simulink model "nmm2DFullBody"  (R2015b)
settings: Solver=ode23s  StartTime=0.0  StopTime=13  FixedStep=1e-3  MaxStep=ts_max  RelTol=1e-3  AbsTol=1e-4
InitFcn:
  | addpath('../lib');
  | addpath('./init_script');
  | nms_model_MechInit
  | nms_model_ControlInit
StopFcn:
  | mRFX = struct;
  | 
  | mRFX.RStance = DataFromModel.Data(:,2)
  | mRFX.RGRF_AP = DataFromModel.Data(:,24)
  | mRFX.RGRF_VT = DataFromModel.Data(:,22)
  | mRFX.RAnkleAngle = DataFromModel.Data(:,8)
  | mRFX.RKneeAngle = DataFromModel.Data(:,7)
  | mRFX.RHipAngle = DataFromModel.Data(:,6)
  | mRFX.RAnkleTorque = DataFromModel.Data(:,20)
  | mRFX.RKneeTorque = DataFromModel.Data(:,19)
  | mRFX.RHipTorque = DataFromModel.Data(:,18)
  | 
  | mRFX.RMuscleGLU = DataFromModel.Data(:,32)
  | mRFX.RMuscleHF = DataFromModel.Data(:,33)
  | mRFX.RMuscleHAM = DataFromModel.Data(:,34)
  | mRFX.RMuscleVAS = DataFromModel.Data(:,35)
  | mRFX.RMuscleGAS = DataFromModel.Data(:,36)
  | mRFX.RMuscleSOL = DataFromModel.Data(:,37)
  | mRFX.RMuscleTA = DataFromModel.Data(:,38)
  | 
  | mRFX.LStance = DataFromModel.Data(:,1)
  | mRFX.LGRF_AP = DataFromModel.Data(:,23)
  | mRFX.LGRF_VT = DataFromModel.Data(:,21)
  | mRFX.LAnkleAngle = DataFromModel.Data(:,5)
  | mRFX.LKneeAngle = DataFromModel.Data(:,4)
  | mRFX.LHipAngle = DataFromModel.Data(:,3)
  | mRFX.LAnkleTorque = DataFromModel.Data(:,17)
  | mRFX.LKneeTorque = DataFromModel.Data(:,16)
  | mRFX.LHipTorque = DataFromModel.Data(:,15)
  | 
  | mRFX.LMuscleGLU = DataFromModel.Data(:,25)
  | mRFX.LMuscleHF = DataFromModel.Data(:,26)
  | mRFX.LMuscleHAM = DataFromModel.Data(:,27)
  | mRFX.LMuscleVAS = DataFromModel.Data(:,28)
  | mRFX.LMuscleGAS = DataFromModel.Data(:,29)
  | mRFX.LMuscleSOL = DataFromModel.Data(:,30)
  | mRFX.LMuscleTA = DataFromModel.Data(:,31)
values from neighbouring files (symbols this model uses):
  c = load('struct_mRFX_HAM_symetric_feedback.mat')    [Ex2b.m]
undefined symbols (not defined in the file or in its folder): alphaFmGas, alphaFmGlu, alphaFmHam, alphaFmSol, alphaFmVas, alphaLceHam, alphaLceHfl, alphaLceTa, alphaLceTa1, Amp, amp_var, c_jointstop, D12_F, D12_S, D12_T, D13_F, D1G_F, D1G_HAT, D1G_S, D1G_T, DeltaThRef, eref, FmaxGAS, FmaxGLU, FmaxHAM, FmaxHFL, FmaxSOL, FmaxTA, FmaxVAS, freq, freq_var, GainDeltaTheta, GainGAS, GainGLU, GainHAM, GainHAMHFL, GainHFL, GainKneOverExt, GainSOL, GainSOLTA, GainTA, GainVAS, In_F, In_HAT, In_S, In_T, K, k_gx, k_gy, k_pressure, K_swing, LceOffsetHAM, LceOffsetHFL, LceOffsetTA, LongDelay, loptGAS, loptGLU, loptHAM, loptHFL, loptSOL ... (+82)
libraries: nmc x77, mblibv1 x60, simulink x33, simulink_extras x18
(part 4 of 8)

== system nmm2DFullBody/Full Body Control (created using the nmc library)/Left Side/HFL&HAM Muscles/HAM Actuation  ==
  note: HAM Actuation
  phiHip : Inport
  phiKnee : Inport  Port=2
  StimHam : Inport  Port=3
  " HAM Muscle Spindles" : Gain  Gain=1/loptHAM
  " HAM Fm loop delay" : TransportDelay  DelayTime=ShortDelay
  " HAM Link" : Subsystem
  HAM : Subsystem
  HAM Golgi Tendon Organs : Gain
  HAM Lce loop delay : TransportDelay  DelayTime=ShortDelay
  Mux1 : Mux  Inputs=5
  Product8 : Product  RndMeth=Zero
  Product9 : Product  RndMeth=Zero
  Saturation7 : Saturate  UpperLimit=inf  LowerLimit=0  ZeroCross=off
  Stimulation Bias7 : Constant  Value=LceOffsetHAM
  Subsystem3 : nmc/Subsystem4  GotoTag=LEFT_HAM_FORCE  GotoTag2=LEFT_HAM_FORCE_LOG  GotoTag3=LEFT_HAM_FORCE_NOISE_LOG
  Subsystem5 : nmc/Subsystem4  GotoTag=LEFT_HAM_STIM  GotoTag2=LEFT_HAM_STIM_LOG  GotoTag3=LEFT_HAM_STIM_NOISE_LOG
  Subsystem6 : nmc/Subsystem4  GotoTag=LEFT_HAM_LENGTH  GotoTag2=LEFT_HAM_LENGTH_LOG  GotoTag3=LEFT_HAM_LENGTH_NOISE_LOG
  Subsystem7 : nmc/Subsystem4  GotoTag=LEFT_HAM_VELOCITY  GotoTag2=LEFT_HAM_VELOCITY_LOG  GotoTag3=LEFT_HAM_VELOCITY_NOISE_LOG
  Subsystem8 : nmc/Subsystem4  GotoTag=LEFT_HAM_GOLGI  GotoTag2=LEFT_HAM_GOLGI_LOG  GotoTag3=LEFT_HAM_GOLGI_NOISE_LOG
  Sum26 : Sum  Inputs=-+|  SaturateOnIntegerOverflow=on  InputSameDT=on  OutDataTypeStr=Inherit: Same as first input
  Terminator1 : Terminator
  TauHamHip : Outport
  TauHamKnee : Outport  Port=2
  LceHam : Outport  Port=3
  FmHam : Outport  Port=4
  wires:
  phiKnee/1 -> " HAM Link"/2(phi23 [rad])
  HAM/1(Fmtc) -> Subsystem3/1
  HAM/2(Lce) -> Subsystem6/1
  " HAM Link"/2(lever34 [m]) -> Product8/2
  " HAM Link"/3(lever23 [m]) -> Product9/2
  phiHip/1 -> " HAM Link"/1(phi34 [rad])
  HAM/5(A) -> Mux1/5
  Product8/1 -> TauHamHip/1
  HAM Golgi Tendon Organs/1 -> " HAM Fm loop delay"/1
  " HAM Muscle Spindles"/1 -> Sum26/2
  Sum26/1 -> Saturation7/1
  Mux1/1 -> Terminator1/1
  HAM/4(Lse) -> Mux1/4
  HAM/3(Vce) -> Subsystem7/1
  Stimulation Bias7/1 -> Sum26/1
  Product9/1 -> TauHamKnee/1
  StimHam/1 -> Subsystem5/1
  Saturation7/1 -> HAM Lce loop delay/1
  HAM Lce loop delay/1 -> LceHam/1
  " HAM Fm loop delay"/1 -> FmHam/1
  Subsystem3/1 -> Mux1/1, Subsystem8/1, Product9/1, Product8/1
  Subsystem6/1 -> " HAM Muscle Spindles"/1, Mux1/2
  Subsystem7/1 -> Mux1/3
  " HAM Link"/1(lmtu [m]) -> HAM/2(lmtc [m])
  Subsystem5/1 -> HAM/1(STIM)
  Subsystem8/1 -> HAM Golgi Tendon Organs/1

== system nmm2DFullBody/Full Body Control (created using the nmc library)/Left Side/HFL&HAM Muscles/HFL Actuation ==
  note: HFL Actuation
  phiHip : Inport
  StimHFL : Inport  Port=2
  " HFL" : Subsystem
  " HFL Muscle Spindles" : Gain  Gain=1/loptHFL
  " HFL Link" : Subsystem
  Gain : Gain  Gain=-1
  HFL Lce loop delay : TransportDelay  DelayTime=ShortDelay
  Mux10 : Mux  Inputs=5
  Product7 : Product  RndMeth=Zero
  Saturation5 : Saturate  UpperLimit=inf  LowerLimit=0  ZeroCross=off
  Stimulation Bias5 : Constant  Value=LceOffsetHFL
  Subsystem3 : nmc/Subsystem4  GotoTag=LEFT_HF_FORCE  GotoTag2=LEFT_HF_FORCE_LOG  GotoTag3=LEFT_HF_FORCE_NOISE_LOG
  Subsystem5 : nmc/Subsystem4  GotoTag=LEFT_HF_STIM  GotoTag2=LEFT_HF_STIM_LOG  GotoTag3=LEFT_HF_STIM_NOISE_LOG
  Subsystem6 : nmc/Subsystem4  GotoTag=LEFT_HF_LENGTH  GotoTag2=LEFT_HF_LENGTH_LOG  GotoTag3=LEFT_HF_LENGTH_NOISE_LOG
  Subsystem7 : nmc/Subsystem4  GotoTag=LEFT_HF_VELOCITY  GotoTag2=LEFT_HF_VELOCITY_LOG  GotoTag3=LEFT_HF_VELOCITY_NOISE_LOG
  Sum24 : Sum  Inputs=-+|  SaturateOnIntegerOverflow=on  InputSameDT=on  OutDataTypeStr=Inherit: Same as first input
  Terminator10 : Terminator
  TauHFL : Outport
  LceHFL : Outport  Port=2
  wires:
  Stimulation Bias5/1 -> Sum24/1
  " HFL"/1(Fmtc) -> Subsystem3/1
  " HFL"/2(Lce) -> Subsystem6/1
  " HFL Link"/1(lmtu [m]) -> " HFL"/2(lmtc [m])
  " HFL"/5(A) -> Mux10/5
  " HFL Link"/2(lever [m]) -> Product7/1
  " HFL Muscle Spindles"/1 -> Sum24/2
  Sum24/1 -> Saturation5/1
  Saturation5/1 -> HFL Lce loop delay/1
  Mux10/1 -> Terminator10/1
  " HFL"/4(Lse) -> Mux10/4
  " HFL"/3(Vce) -> Subsystem7/1
  phiHip/1 -> " HFL Link"/1(phi34 [rad])
  StimHFL/1 -> Subsystem5/1
  Product7/1 -> Gain/1
  Gain/1 -> TauHFL/1
  HFL Lce loop delay/1 -> LceHFL/1
  Subsystem5/1 -> " HFL"/1(STIM)
  Subsystem6/1 -> " HFL Muscle Spindles"/1, Mux10/2
  Subsystem7/1 -> Mux10/3
  Subsystem3/1 -> Product7/2, Mux10/1

== system nmm2DFullBody/Full Body Control (created using the nmc library)/Left Side/HFL&HAM Muscles/HFL&HAM Control ==
  note: HFL with HAM Control
  LceHFL : Inport
  LceHam : Inport  Port=2
  FmHam : Inport  Port=3
  Theta : Inport  Port=4
  dTheta : Inport  Port=5
  CLdxThigh : Inport  Port=6
  OLonCL : Inport  Port=7
  StanceSwing : Inport  Port=8
  "ANMC STIM " : Concatenate  NumInputs=1
  ANMC STIM 1 : Concatenate  NumInputs=1
  Demux : Demux  Outputs=2
  Logical Operator : Logic  Operator=NOT  AllPortsSameDT=off  OutDataTypeStr=boolean
  Mux1 : Mux  Inputs=2
  Mux2 : Mux  Inputs=2
  Saturation17 : Saturate  UpperLimit=1  LowerLimit=0.01  ZeroCross=off
  Stance Phase : Subsystem  TreatAsAtomicUnit=on
  Sum18 : Sum
  Swing Phase : Subsystem  TreatAsAtomicUnit=on
  StimHFL : Outport
  StimHAM : Outport  Port=2
  wires:
  Logical Operator/1 -> Swing Phase/Enable
  Theta/1 -> Stance Phase/1(Theta)
  dTheta/1 -> Stance Phase/2(dTheta [rad/s])
  Swing Phase/1(StimHFL) -> Mux1/1
  LceHam/1 -> Swing Phase/3(LceHAM)
  FmHam/1 -> Swing Phase/4(FmHAM)
  Stance Phase/3(Delta_Theta) -> Swing Phase/1(Delta_Theta)
  CLdxThigh/1 -> Stance Phase/3(CLdxThigh [N])
  Stance Phase/1(StimHFL) -> Mux2/1
  Stance Phase/2(StimHAM) -> Mux2/2
  LceHFL/1 -> Swing Phase/2(LceHFL)
  StanceSwing/1 -> Stance Phase/Enable, Logical Operator/1
  Sum18/1 -> Saturation17/1
  Saturation17/1 -> Demux/1
  Mux2/1 -> Sum18/1
  Mux1/1 -> Sum18/2
  Swing Phase/2(StimHAM) -> Mux1/2
  OLonCL/1 -> Stance Phase/4(OLonCL)
  Demux/2 -> ANMC STIM 1/1
  Demux/1 -> "ANMC STIM "/1
  "ANMC STIM "/1 -> StimHFL/1
  ANMC STIM 1/1 -> StimHAM/1

== system nmm2DFullBody/Full Body Control (created using the nmc library)/Left Side/HipJoint left/Hip Joint Limits ==
  note: Hip Joint Limits
  phi [rad] : Inport
  dphi [rad/s] : Inport  Port=2
  Gain2 : Gain  Gain=-1
  Gain3 : Gain  Gain=c_jointstop
  Gain4 : Gain  Gain=1/w_max_jointstop
  Limit Hip Range : simulink/Logic and Bit Operations/Interval Test  IntervalClosedRight=on  uplimit=phi34_UpLimit + 30*pi/180  IntervalClosedLeft=on  lowlimit=10*pi/180  OutDataTypeStr=boolean
  Logical Operator3 : Logic  Operator=NOT  AllPortsSameDT=off  OutDataTypeStr=boolean
  Mux3 : Mux  Inputs=2
  Overextension Torque : Fcn  Expr="- u(1)  *  (1-u(2)) * (u(2)<1) * (u(1)>0)"
  Stop Simulation1 : Stop
  Sum : Sum  Inputs=|+-
  overextension angle : Constant  Value=phi34_UpLimit
  M_stop [Nm] : Outport
  wires:
  Mux3/1 -> Overextension Torque/1
  Gain3/1 -> Mux3/1
  dphi [rad/s]/1 -> Gain4/1
  overextension angle/1 -> Sum/2
  phi [rad]/1 -> Sum/1, Limit Hip Range/1
  Sum/1 -> Gain3/1
  Gain4/1 -> Gain2/1
  Gain2/1 -> Mux3/2
  Overextension Torque/1 -> M_stop [Nm]/1
  Limit Hip Range/1 -> Logical Operator3/1
  Logical Operator3/1 -> Stop Simulation1/1

== system nmm2DFullBody/Full Body Control (created using the nmc library)/Left Side/KneeJoint left/Knee Joint Limits ==
  note: Knee Joint Limits
  phi [rad] : Inport
  dphi [rad/s] : Inport  Port=2
  Gain2 : Gain  Gain=-1
  Gain3 : Gain  Gain=c_jointstop
  Gain4 : Gain  Gain=1/w_max_jointstop
  Limit Knee Range : simulink/Logic and Bit Operations/Interval Test  IntervalClosedRight=on  uplimit=185*pi/180  IntervalClosedLeft=on  lowlimit=40*pi/180  OutDataTypeStr=boolean
  Logical Operator3 : Logic  Operator=NOT  AllPortsSameDT=off  OutDataTypeStr=boolean
  Mux3 : Mux  Inputs=2
  Overextension Torque : Fcn  Expr="- u(1)  *  (1-u(2)) * (u(2)<1) * (u(1)>0)"
  Stop Simulation1 : Stop
  Sum : Sum  Inputs=|+-
  overextension angle : Constant  Value=phi23_UpLimit
  M_stop [Nm] : Outport
  wires:
  Mux3/1 -> Overextension Torque/1
  Gain3/1 -> Mux3/1
  dphi [rad/s]/1 -> Gain4/1
  overextension angle/1 -> Sum/2
  phi [rad]/1 -> Sum/1, Limit Knee Range/1
  Sum/1 -> Gain3/1
  Gain4/1 -> Gain2/1
  Gain2/1 -> Mux3/2
  Overextension Torque/1 -> M_stop [Nm]/1
  Limit Knee Range/1 -> Logical Operator3/1
  Logical Operator3/1 -> Stop Simulation1/1

== system nmm2DFullBody/Full Body Control (created using the nmc library)/Left Side/SOL&TA Muscles/SOL Actuation ==
  note: SOL Actuation
  phiAnkle : Inport
  StimSOL : Inport  Port=2
  " SOL" : Subsystem
  " SOL Golgi Tendon Organs" : Gain
  Mux3 : Mux  Inputs=5
  Product : Product  RndMeth=Zero
  SOL Link : Subsystem
  SOL loop delay : TransportDelay  DelayTime=LongDelay
  Subsystem3 : nmc/Subsystem4  GotoTag=LEFT_SOL_FORCE  GotoTag2=LEFT_SOL_FORCE_LOG  GotoTag3=LEFT_SOL_FORCE_NOISE_LOG
  Subsystem5 : nmc/Subsystem4  GotoTag=LEFT_SOL_STIM  GotoTag2=LEFT_SOL_STIM_LOG  GotoTag3=LEFT_SOL_STIM_NOISE_LOG
  Subsystem6 : nmc/Subsystem4  GotoTag=LEFT_SOL_LENGTH  GotoTag2=LEFT_SOL_LENGTH_LOG  GotoTag3=LEFT_SOL_LENGTH_NOISE_LOG
  Subsystem7 : nmc/Subsystem4  GotoTag=LEFT_SOL_VELOCITY  GotoTag2=LEFT_SOL_VELOCITY_LOG  GotoTag3=LEFT_SOL_VELOCITY_NOISE_LOG
  Subsystem8 : nmc/Subsystem4  GotoTag=LEFT_SOL_GOLGI  GotoTag2=LEFT_SOL_GOLGI_LOG  GotoTag3=LEFT_SOL_GOLGI_NOISE_LOG
  Terminator3 : Terminator
  TauSOL : Outport
  FmSOL : Outport  Port=2
  wires:
  " SOL"/1(Fmtc) -> Subsystem3/1
  SOL Link/1(lmtc [m]) -> " SOL"/2(lmtc [m])
  SOL Link/2(lever [m]) -> Product/1
  Product/1 -> TauSOL/1
  " SOL"/5(A) -> Mux3/5
  Mux3/1 -> Terminator3/1
  " SOL"/2(Lce) -> Subsystem6/1
  " SOL"/3(Vce) -> Subsystem7/1
  " SOL"/4(Lse) -> Mux3/4
  phiAnkle/1 -> SOL Link/1(phi12 [rad])
  StimSOL/1 -> Subsystem5/1
  " SOL Golgi Tendon Organs"/1 -> SOL loop delay/1
  SOL loop delay/1 -> FmSOL/1
  Subsystem5/1 -> " SOL"/1(STIM)
  Subsystem3/1 -> Mux3/1, Product/2, Subsystem8/1
  Subsystem6/1 -> Mux3/2
  Subsystem7/1 -> Mux3/3
  Subsystem8/1 -> " SOL Golgi Tendon Organs"/1

== system nmm2DFullBody/Full Body Control (created using the nmc library)/Left Side/SOL&TA Muscles/SOL&TA Control ==
  note: SOL with TA Control
  LceTA : Inport
  FmSOL : Inport  Port=2
  StanceSwing : Inport  Port=3
  " Stance Phase" : Subsystem  TreatAsAtomicUnit=on
  "ANMC STIM " : Concatenate  NumInputs=1
  ANMC STIM 1 : Concatenate  NumInputs=1
  Demux : Demux  Outputs=2
  Logical Operator : Logic  Operator=NOT  AllPortsSameDT=off  OutDataTypeStr=boolean
  Mux1 : Mux  Inputs=2
  Mux2 : Mux  Inputs=2
  Saturation17 : Saturate  UpperLimit=1  LowerLimit=0.01  ZeroCross=off
  Sum18 : Sum
  Swing Phase : Subsystem  TreatAsAtomicUnit=on
  StimTA : Outport
  StimSOL : Outport  Port=2
  wires:
  Logical Operator/1 -> Swing Phase/Enable
  FmSOL/1 -> " Stance Phase"/1(FmSOL)
  StanceSwing/1 -> " Stance Phase"/Enable, Logical Operator/1
  LceTA/1 -> Swing Phase/1(LceTA), " Stance Phase"/2(LceTA)
  Swing Phase/1(StimTA) -> Mux1/1
  " Stance Phase"/1(StimTA) -> Mux2/1
  " Stance Phase"/2(StimSOL) -> Mux2/2
  Sum18/1 -> Saturation17/1
  Saturation17/1 -> Demux/1
  Mux2/1 -> Sum18/1
  Mux1/1 -> Sum18/2
  Swing Phase/2(StimSOL) -> Mux1/2
  Demux/2 -> ANMC STIM 1/1
  Demux/1 -> "ANMC STIM "/1
  "ANMC STIM "/1 -> StimTA/1
  ANMC STIM 1/1 -> StimSOL/1

== system nmm2DFullBody/Full Body Control (created using the nmc library)/Left Side/SOL&TA Muscles/TA Actuation ==
  note: TA Actuation
  phiAnkle : Inport
  StimTA : Inport  Port=2
  " TA Muscle Spindles" : Gain  Gain=1/loptTA
  " TA loop delay" : TransportDelay  DelayTime=LongDelay
  Gain : Gain  Gain=-1
  Mux8 : Mux  Inputs=5
  Product1 : Product  RndMeth=Zero
  Saturation2 : Saturate  UpperLimit=inf  LowerLimit=0  ZeroCross=off
  Stimulation Bias3 : Constant  Value=LceOffsetTA
  Subsystem3 : nmc/Subsystem4  GotoTag=LEFT_TA_FORCE  GotoTag2=LEFT_TA_FORCE_LOG  GotoTag3=LEFT_TA_FORCE_NOISE_LOG
  Subsystem5 : nmc/Subsystem4  GotoTag=LEFT_TA_STIM  GotoTag2=LEFT_TA_STIM_LOG  GotoTag3=LEFT_TA_STIM_NOISE_LOG
  Subsystem6 : nmc/Subsystem4  GotoTag=LEFT_TA_LENGTH  GotoTag2=LEFT_TA_LENGTH_LOG  GotoTag3=LEFT_TA_LENGTH_NOISE_LOG
  Subsystem7 : nmc/Subsystem4  GotoTag=LEFT_TA_VELOCITY  GotoTag2=LEFT_TA_VELOCITY_LOG  GotoTag3=LEFT_TA_VELOCITY_NOISE_LOG
  Sum21 : Sum  Inputs=-+|  SaturateOnIntegerOverflow=on  InputSameDT=on  OutDataTypeStr=Inherit: Same as first input
  TA : Subsystem
  TA Link : Subsystem
  Terminator8 : Terminator
  LceTA : Outport
  TauTa : Outport  Port=2
  wires:
  TA/1(Fmtc) -> Subsystem3/1
  TA/2(Lce) -> Subsystem6/1
  TA/5(A) -> Mux8/5
  TA Link/1(lmtc [m]) -> TA/2(lmtc [m])
  TA Link/2(lever [m]) -> Product1/2
  " TA Muscle Spindles"/1 -> Sum21/2
  Sum21/1 -> Saturation2/1
  Mux8/1 -> Terminator8/1
  TA/4(Lse) -> Mux8/4
  TA/3(Vce) -> Subsystem7/1
  phiAnkle/1 -> TA Link/1(phi12 [rad])
  Stimulation Bias3/1 -> Sum21/1
  Saturation2/1 -> " TA loop delay"/1
  Product1/1 -> Gain/1
  StimTA/1 -> Subsystem5/1
  " TA loop delay"/1 -> LceTA/1
  Gain/1 -> TauTa/1
  Subsystem5/1 -> TA/1(STIM)
  Subsystem3/1 -> Product1/1, Mux8/1
  Subsystem6/1 -> " TA Muscle Spindles"/1, Mux8/2
  Subsystem7/1 -> Mux8/3

== system nmm2DFullBody/Full Body Control (created using the nmc library)/Left Side/VAS Muscle/VAS Actuation  ==
  note: VAS Actuation
  phiKnee : Inport
  StimVas : Inport  Port=2
  " VAS Golgi Tendon Organs" : Gain
  Gain : Gain  Gain=-1
  Mux9 : Mux  Inputs=5
  Product4 : Product  RndMeth=Zero
  Subsystem3 : nmc/Subsystem4  GotoTag=LEFT_VAS_FORCE  GotoTag2=LEFT_VAS_FORCE_LOG  GotoTag3=LEFT_VAS_FORCE_NOISE_LOG
  Subsystem5 : nmc/Subsystem4  GotoTag=LEFT_VAS_STIM  GotoTag2=LEFT_VAS_STIM_LOG  GotoTag3=LEFT_VAS_STIM_NOISE_LOG
  Subsystem6 : nmc/Subsystem4  GotoTag=LEFT_VAS_LENGTH  GotoTag2=LEFT_VAS_LENGTH_LOG  GotoTag3=LEFT_VAS_LENGTH_NOISE_LOG
  Subsystem7 : nmc/Subsystem4  GotoTag=LEFT_VAS_VELOCITY  GotoTag2=LEFT_VAS_VELOCITY_LOG  GotoTag3=LEFT_VAS_VELOCITY_NOISE_LOG
  Subsystem8 : nmc/Subsystem4  GotoTag=LEFT_VAS_GOLGI  GotoTag2=LEFT_VAS_GOLGI_LOG  GotoTag3=LEFT_VAS_GOLGI_NOISE_LOG
  Terminator9 : Terminator
  VAS : Subsystem
  VAS Link : Subsystem
  VAS loop delay : TransportDelay  DelayTime=MidDelay
  TauVas : Outport
  FmVas : Outport  Port=2
  wires:
  Product4/1 -> Gain/1
  VAS/5(A) -> Mux9/5
  VAS/1(Fmtc) -> Subsystem3/1
  VAS Link/2(lever [m]) -> Product4/1
  Mux9/1 -> Terminator9/1
  VAS/4(Lse) -> Mux9/4
  VAS/3(Vce) -> Subsystem7/1
  VAS/2(Lce) -> Subsystem6/1
  phiKnee/1 -> VAS Link/1(phi23 [rad])
  StimVas/1 -> Subsystem5/1
  Gain/1 -> TauVas/1
  " VAS Golgi Tendon Organs"/1 -> VAS loop delay/1
  VAS loop delay/1 -> FmVas/1
  VAS Link/1(lmtu [m]) -> VAS/2(lmtc [m])
  Subsystem3/1 -> Subsystem8/1, Product4/2, Mux9/1
  Subsystem6/1 -> Mux9/2
  Subsystem7/1 -> Mux9/3
  Subsystem5/1 -> VAS/1(STIM)
  Subsystem8/1 -> " VAS Golgi Tendon Organs"/1

== system nmm2DFullBody/Full Body Control (created using the nmc library)/Left Side/VAS Muscle/VAS Control ==
  note: VAS Control
  FmVAS : Inport
  OLdxThigh : Inport  Port=2
  OLonCL : Inport  Port=3
  CLKneeState : Inport  Port=4
  StanceSwing : Inport  Port=5
  " Swing Phase" : Subsystem  TreatAsAtomicUnit=on
  "ANMC STIM " : Concatenate  NumInputs=1
  Logical Operator : Logic  Operator=NOT  AllPortsSameDT=off  OutDataTypeStr=boolean
  Saturation17 : Saturate  UpperLimit=1  LowerLimit=0.01  ZeroCross=off
  Stance Phase : Subsystem  TreatAsAtomicUnit=on
  Sum18 : Sum
  StimVAS : Outport
  wires:
  Logical Operator/1 -> " Swing Phase"/Enable
  FmVAS/1 -> Stance Phase/4(FmVAS)
  StanceSwing/1 -> Logical Operator/1, Stance Phase/Enable
  " Swing Phase"/1(StimVAS) -> Sum18/2
  Sum18/1 -> Saturation17/1
  Saturation17/1 -> "ANMC STIM "/1
  Stance Phase/1(StimVAS) -> Sum18/1
  OLdxThigh/1 -> Stance Phase/3(OLdxThigh [N])
  OLonCL/1 -> Stance Phase/2(OLonCL)
  CLKneeState/1 -> Stance Phase/1(CLKneeState)
  "ANMC STIM "/1 -> StimVAS/1

== system nmm2DFullBody/Full Body Control (created using the nmc library)/Right Side/GAS Muscle/GAS Actuation  ==
  note: GAS Actuation
  phiKnee : Inport
  phiAnkle : Inport  Port=2
  StimGas : Inport  Port=3
  " GAS" : Subsystem
  " GAS Golgi Tendon Organs" : Gain
  GAS Link : Subsystem
  GAS loop delay : TransportDelay  DelayTime=LongDelay
  Mux2 : Mux  Inputs=5
  Product2 : Product  RndMeth=Zero
  Product3 : Product  RndMeth=Zero
  Subsystem3 : nmc/Subsystem4  GotoTag=RIGHT_GAS_FORCE  GotoTag2=RIGHT_GAS_FORCE_LOG  GotoTag3=RIGHT_GAS_FORCE_NOISE_LOG
  Subsystem5 : nmc/Subsystem4  GotoTag=RIGHT_GAS_STIM  GotoTag2=RIGHT_GAS_STIM_LOG  GotoTag3=RIGHT_GAS_STIM_NOISE_LOG
  Subsystem6 : nmc/Subsystem4  GotoTag=RIGHT_GAS_LENGTH  GotoTag2=RIGHT_GAS_LENGTH_LOG  GotoTag3=RIGHT_GAS_LENGTH_NOISE_LOG
  Subsystem7 : nmc/Subsystem4  GotoTag=RIGHT_GAS_VELOCITY  GotoTag2=RIGHT_GAS_VELOCITY_LOG  GotoTag3=RIGHT_GAS_VELOCITY_NOISE_LOG
  Subsystem8 : nmc/Subsystem4  GotoTag=RIGHT_GAS_GOLGI  GotoTag2=RIGHT_GAS_GOLGI_LOG  GotoTag3=RIGHT_GAS_GOLGI_NOISE_LOG
  Terminator2 : Terminator
  TauGasKnee : Outport
  TauGasAnkle : Outport  Port=2
  FmGas : Outport  Port=3
  wires:
  " GAS"/1(Fmtc) -> Subsystem3/1
  GAS Link/3(lever12 [m]) -> Product2/2
  GAS Link/2(lever23 [m]) -> Product3/2
  GAS Link/1(lmtu [m]) -> " GAS"/2(lmtc [m])
  Product3/1 -> TauGasKnee/1
  " GAS"/5(A) -> Mux2/5
  Mux2/1 -> Terminator2/1
  " GAS"/4(Lse) -> Mux2/4
  " GAS"/3(Vce) -> Subsystem7/1
  " GAS"/2(Lce) -> Subsystem6/1
  phiKnee/1 -> GAS Link/1(phi23 [rad])
  phiAnkle/1 -> GAS Link/2(phi12 [rad])
  StimGas/1 -> Subsystem5/1
  Product2/1 -> TauGasAnkle/1
  " GAS Golgi Tendon Organs"/1 -> GAS loop delay/1
  GAS loop delay/1 -> FmGas/1
  Subsystem5/1 -> " GAS"/1(STIM)
  Subsystem3/1 -> Mux2/1, Product2/1, Product3/1, Subsystem8/1
  Subsystem6/1 -> Mux2/2
  Subsystem7/1 -> Mux2/3
  Subsystem8/1 -> " GAS Golgi Tendon Organs"/1

== system nmm2DFullBody/Full Body Control (created using the nmc library)/Right Side/GAS Muscle/GAS Control ==
  note: GAS sControl
  FmGAS : Inport
  StanceSwing : Inport  Port=2
  " Swing Phase" : Subsystem  TreatAsAtomicUnit=on
  "ANMC STIM " : Concatenate  NumInputs=1
  Logical Operator : Logic  Operator=NOT  AllPortsSameDT=off  OutDataTypeStr=boolean
  Saturation17 : Saturate  UpperLimit=1  LowerLimit=0.01  ZeroCross=off
  Stance Phase : Subsystem  TreatAsAtomicUnit=on
  Sum18 : Sum
  StimGAS : Outport
  wires:
  Logical Operator/1 -> " Swing Phase"/Enable
  FmGAS/1 -> Stance Phase/1(FmGAS)
  StanceSwing/1 -> Logical Operator/1, Stance Phase/Enable
  " Swing Phase"/1(StimGAS) -> Sum18/2
  Sum18/1 -> Saturation17/1
  Saturation17/1 -> "ANMC STIM "/1
  Stance Phase/1(StimGAS) -> Sum18/1
  "ANMC STIM "/1 -> StimGAS/1

== system nmm2DFullBody/Full Body Control (created using the nmc library)/Right Side/GLU Muscle/GLU Actuation ==
  note: GLU Actuation
  phiHip : Inport
  StimGlu : Inport  Port=2
  " GLU" : Subsystem
  " GLU Fm loop delay" : TransportDelay  DelayTime=ShortDelay
  GLU Golgi Tendon Organs : Gain
  GLU Link : Subsystem
  Mux : Mux  Inputs=5
  Product6 : Product  RndMeth=Zero
  Subsystem3 : nmc/Subsystem4  GotoTag=RIGHT_GLU_FORCE  GotoTag2=RIGHT_GLU_FORCE_LOG  GotoTag3=RIGHT_GLU_FORCE_NOISE_LOG
  Subsystem5 : nmc/Subsystem4  GotoTag=RIGHT_GLU_STIM  GotoTag2=RIGHT_GLU_STIM_LOG  GotoTag3=RIGHT_GLU_STIM_NOISE_LOG
  Subsystem6 : nmc/Subsystem4  GotoTag=RIGHT_GLU_LENGTH  GotoTag2=RIGHT_GLU_LENGTH_LOG  GotoTag3=RIGHT_GLU_LENGTH_NOISE_LOG
  Subsystem7 : nmc/Subsystem4  GotoTag=RIGHT_GLU_VELOCITY  GotoTag2=RIGHT_GLU_VELOCITY_LOG  GotoTag3=RIGHT_GLU_VELOCITY_NOISE_LOG
  Subsystem8 : nmc/Subsystem4  GotoTag=RIGHT_GLU_GOLGI  GotoTag2=RIGHT_GLU_GOLGI_LOG  GotoTag3=RIGHT_GLU_GOLGI_NOISE_LOG
  Terminator : Terminator
  TauGlu : Outport
  FmGlu : Outport  Port=2
  wires:
  " GLU"/1(Fmtc) -> Subsystem3/1
  StimGlu/1 -> Subsystem5/1
  Product6/1 -> TauGlu/1
  GLU Link/1(lmtu [m]) -> " GLU"/2(lmtc [m])
  GLU Link/2(lever [m]) -> Product6/2
  " GLU"/5(A) -> Mux/5
  GLU Golgi Tendon Organs/1 -> " GLU Fm loop delay"/1
  " GLU"/2(Lce) -> Subsystem6/1
  " GLU"/3(Vce) -> Subsystem7/1
  " GLU"/4(Lse) -> Mux/4
  Mux/1 -> Terminator/1
  phiHip/1 -> GLU Link/1(phi34 [rad])
  " GLU Fm loop delay"/1 -> FmGlu/1
  Subsystem5/1 -> " GLU"/1(STIM)
  Subsystem3/1 -> Mux/1, Product6/1, Subsystem8/1
  Subsystem6/1 -> Mux/2
  Subsystem7/1 -> Mux/3
  Subsystem8/1 -> GLU Golgi Tendon Organs/1

== system nmm2DFullBody/Full Body Control (created using the nmc library)/Right Side/GLU Muscle/GLU Control ==
  note: GLU Control
  FmGlu : Inport
  Theta : Inport  Port=2
  dTheta : Inport  Port=3
  CLdxThigh : Inport  Port=4
  OLonCL : Inport  Port=5
  StanceSwing : Inport  Port=6
  " Swing Phase" : Subsystem  TreatAsAtomicUnit=on
  "ANMC STIM " : Concatenate  NumInputs=1
  Logical Operator : Logic  Operator=NOT  AllPortsSameDT=off  OutDataTypeStr=boolean
  Saturation17 : Saturate  UpperLimit=1  LowerLimit=0.01  ZeroCross=off
  Stance Phase : Subsystem  TreatAsAtomicUnit=on
  Sum18 : Sum
  StimGlu : Outport
  wires:
  Logical Operator/1 -> " Swing Phase"/Enable
  " Swing Phase"/1(StimGLU) -> Sum18/2
  FmGlu/1 -> " Swing Phase"/1(FmGLU)
  Sum18/1 -> Saturation17/1
  Saturation17/1 -> "ANMC STIM "/1
  dTheta/1 -> Stance Phase/2(dTheta [rad/s])
  Theta/1 -> Stance Phase/1(Theta)
  Stance Phase/1(StimGLU) -> Sum18/1
  CLdxThigh/1 -> Stance Phase/3(CLdxThigh [N])
  OLonCL/1 -> Stance Phase/4(OLonCL)
  StanceSwing/1 -> Logical Operator/1, Stance Phase/Enable
  "ANMC STIM "/1 -> StimGlu/1

== system nmm2DFullBody/Full Body Control (created using the nmc library)/Right Side/HFL&HAM Muscles/HAM Actuation  ==
  note: HAM Actuation
  phiHip : Inport
  phiKnee : Inport  Port=2
  StimHam : Inport  Port=3
  " HAM Muscle Spindles" : Gain  Gain=1/loptHAM
  " HAM Fm loop delay" : TransportDelay  DelayTime=ShortDelay
  " HAM Link" : Subsystem
  HAM : Subsystem
  HAM Golgi Tendon Organs : Gain
  HAM Lce loop delay : TransportDelay  DelayTime=ShortDelay
  Mux1 : Mux  Inputs=5
  Product8 : Product  RndMeth=Zero
  Product9 : Product  RndMeth=Zero
  Saturation7 : Saturate  UpperLimit=inf  LowerLimit=0  ZeroCross=off
  Stimulation Bias7 : Constant  Value=LceOffsetHAM
  Subsystem3 : nmc/Subsystem4  GotoTag=RIGHT_HAM_FORCE  GotoTag2=RIGHT_HAM_FORCE_LOG  GotoTag3=RIGHT_HAM_FORCE_NOISE_LOG
  Subsystem5 : nmc/Subsystem4  GotoTag=RIGHT_HAM_STIM  GotoTag2=RIGHT_HAM_STIM_LOG  GotoTag3=RIGHT_HAM_STIM_NOISE_LOG
  Subsystem6 : nmc/Subsystem4  GotoTag=RIGHT_HAM_LENGTH  GotoTag2=RIGHT_HAM_LENGTH_LOG  GotoTag3=RIGHT_HAM_LENGTH_NOISE_LOG
  Subsystem7 : nmc/Subsystem4  GotoTag=RIGHT_HAM_VELOCITY  GotoTag2=RIGHT_HAM_VELOCITY_LOG  GotoTag3=RIGHT_HAM_VELOCITY_NOISE_LOG
  Subsystem8 : nmc/Subsystem4  GotoTag=RIGHT_HAM_GOLGI  GotoTag2=RIGHT_HAM_GOLGI_LOG  GotoTag3=RIGHT_HAM_GOLGI_NOISE_LOG
  Sum26 : Sum  Inputs=-+|  SaturateOnIntegerOverflow=on  InputSameDT=on  OutDataTypeStr=Inherit: Same as first input
  Terminator1 : Terminator
  TauHamHip : Outport
  TauHamKnee : Outport  Port=2
  LceHam : Outport  Port=3
  FmHam : Outport  Port=4
  wires:
  phiKnee/1 -> " HAM Link"/2(phi23 [rad])
  HAM/1(Fmtc) -> Subsystem3/1
  HAM/2(Lce) -> Subsystem6/1
  " HAM Link"/1(lmtu [m]) -> HAM/2(lmtc [m])
  " HAM Link"/2(lever34 [m]) -> Product8/2
  " HAM Link"/3(lever23 [m]) -> Product9/2
  phiHip/1 -> " HAM Link"/1(phi34 [rad])
  HAM/5(A) -> Mux1/5
  Product8/1 -> TauHamHip/1
  HAM Golgi Tendon Organs/1 -> " HAM Fm loop delay"/1
  " HAM Muscle Spindles"/1 -> Sum26/2
  Sum26/1 -> Saturation7/1
  Mux1/1 -> Terminator1/1
  HAM/4(Lse) -> Mux1/4
  HAM/3(Vce) -> Subsystem7/1
  Stimulation Bias7/1 -> Sum26/1
  Product9/1 -> TauHamKnee/1
  StimHam/1 -> Subsystem5/1
  Saturation7/1 -> HAM Lce loop delay/1
  HAM Lce loop delay/1 -> LceHam/1
  " HAM Fm loop delay"/1 -> FmHam/1
  Subsystem5/1 -> HAM/1(STIM)
  Subsystem3/1 -> Mux1/1, Subsystem8/1, Product9/1, Product8/1
  Subsystem6/1 -> " HAM Muscle Spindles"/1, Mux1/2
  Subsystem7/1 -> Mux1/3
  Subsystem8/1 -> HAM Golgi Tendon Organs/1

== system nmm2DFullBody/Full Body Control (created using the nmc library)/Right Side/HFL&HAM Muscles/HFL Actuation ==
  note: HFL Actuation
  phiHip : Inport
  StimHFL : Inport  Port=2
  " HFL" : Subsystem
  " HFL Muscle Spindles" : Gain  Gain=1/loptHFL
  " HFL Link" : Subsystem
  Gain : Gain  Gain=-1
  HFL Lce loop delay : TransportDelay  DelayTime=ShortDelay
  Mux10 : Mux  Inputs=5
  Product7 : Product  RndMeth=Zero
  Saturation5 : Saturate  UpperLimit=inf  LowerLimit=0  ZeroCross=off
  Stimulation Bias5 : Constant  Value=LceOffsetHFL
  Subsystem3 : nmc/Subsystem4  GotoTag=RIGHT_HF_FORCE  GotoTag2=RIGHT_HF_FORCE_LOG  GotoTag3=RIGHT_HF_FORCE_NOISE_LOG
  Subsystem5 : nmc/Subsystem4  GotoTag=RIGHT_HF_STIM  GotoTag2=RIGHT_HF_STIM_LOG  GotoTag3=RIGHT_HF_STIM_NOISE_LOG
  Subsystem6 : nmc/Subsystem4  GotoTag=RIGHT_HF_LENGTH  GotoTag2=RIGHT_HF_LENGTH_LOG  GotoTag3=RIGHT_HF_LENGTH_NOISE_LOG
  Subsystem7 : nmc/Subsystem4  GotoTag=RIGHT_HF_VELOCITY  GotoTag2=RIGHT_HF_VELOCITY_LOG  GotoTag3=RIGHT_HF_VELOCITY_NOISE_LOG
  Sum24 : Sum  Inputs=-+|  SaturateOnIntegerOverflow=on  InputSameDT=on  OutDataTypeStr=Inherit: Same as first input
  Terminator10 : Terminator
  TauHFL : Outport
  LceHFL : Outport  Port=2
  wires:
  Stimulation Bias5/1 -> Sum24/1
  " HFL"/1(Fmtc) -> Subsystem3/1
  " HFL"/2(Lce) -> Subsystem6/1
  " HFL Link"/1(lmtu [m]) -> " HFL"/2(lmtc [m])
  " HFL"/5(A) -> Mux10/5
  " HFL Link"/2(lever [m]) -> Product7/1
  " HFL Muscle Spindles"/1 -> Sum24/2
  Sum24/1 -> Saturation5/1
  Saturation5/1 -> HFL Lce loop delay/1
  Mux10/1 -> Terminator10/1
  " HFL"/4(Lse) -> Mux10/4
  " HFL"/3(Vce) -> Subsystem7/1
  phiHip/1 -> " HFL Link"/1(phi34 [rad])
  StimHFL/1 -> Subsystem5/1
  Product7/1 -> Gain/1
  Gain/1 -> TauHFL/1
  HFL Lce loop delay/1 -> LceHFL/1
  Subsystem5/1 -> " HFL"/1(STIM)
  Subsystem3/1 -> Product7/2, Mux10/1
  Subsystem6/1 -> " HFL Muscle Spindles"/1, Mux10/2
  Subsystem7/1 -> Mux10/3

== system nmm2DFullBody/Full Body Control (created using the nmc library)/Right Side/HFL&HAM Muscles/HFL&HAM Control ==
  note: HFL with HAM Control
  LceHFL : Inport
  LceHam : Inport  Port=2
  FmHam : Inport  Port=3
  Theta : Inport  Port=4
  dTheta : Inport  Port=5
  CLdxThigh : Inport  Port=6
  OLonCL : Inport  Port=7
  StanceSwing : Inport  Port=8
  "ANMC STIM " : Concatenate  NumInputs=1
  ANMC STIM 1 : Concatenate  NumInputs=1
  Demux : Demux  Outputs=2
  Logical Operator : Logic  Operator=NOT  AllPortsSameDT=off  OutDataTypeStr=boolean
  Mux1 : Mux  Inputs=2
  Mux2 : Mux  Inputs=2
  Saturation17 : Saturate  UpperLimit=1  LowerLimit=0.01  ZeroCross=off
  Stance Phase : Subsystem  TreatAsAtomicUnit=on
  Sum18 : Sum
  Swing Phase : Subsystem  TreatAsAtomicUnit=on
  StimHFL : Outport
  StimHAM : Outport  Port=2
  wires:
  Logical Operator/1 -> Swing Phase/Enable
  Theta/1 -> Stance Phase/1(Theta)
  dTheta/1 -> Stance Phase/2(dTheta [rad/s])
  Swing Phase/1(StimHFL) -> Mux1/1
  LceHam/1 -> Swing Phase/3(LceHAM)
  FmHam/1 -> Swing Phase/4(FmHAM)
  Stance Phase/3(Delta_Theta) -> Swing Phase/1(Delta_Theta)
  CLdxThigh/1 -> Stance Phase/3(CLdxThigh [N])
  Stance Phase/1(StimHFL) -> Mux2/1
  Stance Phase/2(StimHAM) -> Mux2/2
  LceHFL/1 -> Swing Phase/2(LceHFL)
  StanceSwing/1 -> Stance Phase/Enable, Logical Operator/1
  Sum18/1 -> Saturation17/1
  Saturation17/1 -> Demux/1
  Mux2/1 -> Sum18/1
  Mux1/1 -> Sum18/2
  Swing Phase/2(StimHAM) -> Mux1/2
  OLonCL/1 -> Stance Phase/4(OLonCL)
  Demux/2 -> ANMC STIM 1/1
  Demux/1 -> "ANMC STIM "/1
  "ANMC STIM "/1 -> StimHFL/1
  ANMC STIM 1/1 -> StimHAM/1

== system nmm2DFullBody/Full Body Control (created using the nmc library)/Right Side/SOL&TA Muscles/SOL Actuation ==
  note: SOL Actuation
  phiAnkle : Inport
  StimSOL : Inport  Port=2
  " SOL" : Subsystem
  " SOL Golgi Tendon Organs" : Gain
  Mux3 : Mux  Inputs=5
  Product : Product  RndMeth=Zero
  SOL Link : Subsystem
  SOL loop delay : TransportDelay  DelayTime=LongDelay
  Subsystem3 : nmc/Subsystem4  GotoTag=RIGHT_SOL_FORCE  GotoTag2=RIGHT_SOL_FORCE_LOG  GotoTag3=RIGHT_SOL_FORCE_NOISE_LOG
  Subsystem5 : nmc/Subsystem4  GotoTag=RIGHT_SOL_STIM  GotoTag2=RIGHT_SOL_STIM_LOG  GotoTag3=RIGHT_SOL_STIM_NOISE_LOG
  Subsystem6 : nmc/Subsystem4  GotoTag=RIGHT_SOL_LENGTH  GotoTag2=RIGHT_SOL_LENGTH_LOG  GotoTag3=RIGHT_SOL_LENGTH_NOISE_LOG
  Subsystem7 : nmc/Subsystem4  GotoTag=RIGHT_SOL_VELOCITY  GotoTag2=RIGHT_SOL_VELOCITY_LOG  GotoTag3=RIGHT_SOL_VELOCITY_NOISE_LOG
  Subsystem8 : nmc/Subsystem4  GotoTag=RIGHT_SOL_GOLGI  GotoTag2=RIGHT_SOL_GOLGI_LOG  GotoTag3=RIGHT_SOL_GOLGI_NOISE_LOG
  Terminator3 : Terminator
  TauSOL : Outport
  FmSOL : Outport  Port=2
  wires:
  " SOL"/1(Fmtc) -> Subsystem3/1
  SOL Link/1(lmtc [m]) -> " SOL"/2(lmtc [m])
  SOL Link/2(lever [m]) -> Product/1
  Product/1 -> TauSOL/1
  " SOL"/5(A) -> Mux3/5
  Mux3/1 -> Terminator3/1
  " SOL"/2(Lce) -> Subsystem6/1
  " SOL"/3(Vce) -> Subsystem7/1
  " SOL"/4(Lse) -> Mux3/4
  phiAnkle/1 -> SOL Link/1(phi12 [rad])
  StimSOL/1 -> Subsystem5/1
  " SOL Golgi Tendon Organs"/1 -> SOL loop delay/1
  SOL loop delay/1 -> FmSOL/1
  Subsystem5/1 -> " SOL"/1(STIM)
  Subsystem3/1 -> Product/2, Subsystem8/1, Mux3/1
  Subsystem6/1 -> Mux3/2
  Subsystem7/1 -> Mux3/3
  Subsystem8/1 -> " SOL Golgi Tendon Organs"/1

== system nmm2DFullBody/Full Body Control (created using the nmc library)/Right Side/SOL&TA Muscles/SOL&TA Control ==
  note: SOL with TA Control
  LceTA : Inport
  FmSOL : Inport  Port=2
  StanceSwing : Inport  Port=3
  " Stance Phase" : Subsystem  TreatAsAtomicUnit=on
  "ANMC STIM " : Concatenate  NumInputs=1
  ANMC STIM 1 : Concatenate  NumInputs=1
  Demux : Demux  Outputs=2
  Logical Operator : Logic  Operator=NOT  AllPortsSameDT=off  OutDataTypeStr=boolean
  Mux1 : Mux  Inputs=2
  Mux2 : Mux  Inputs=2
  Saturation17 : Saturate  UpperLimit=1  LowerLimit=0.01  ZeroCross=off
  Sum18 : Sum
  Swing Phase : Subsystem  TreatAsAtomicUnit=on
  StimTA : Outport
  StimSOL : Outport  Port=2
  wires:
  Logical Operator/1 -> Swing Phase/Enable
  FmSOL/1 -> " Stance Phase"/1(FmSOL)
  StanceSwing/1 -> " Stance Phase"/Enable, Logical Operator/1
  LceTA/1 -> Swing Phase/1(LceTA), " Stance Phase"/2(LceTA)
  Swing Phase/1(StimTA) -> Mux1/1
  " Stance Phase"/1(StimTA) -> Mux2/1
  " Stance Phase"/2(StimSOL) -> Mux2/2
  Sum18/1 -> Saturation17/1
  Saturation17/1 -> Demux/1
  Mux2/1 -> Sum18/1
  Mux1/1 -> Sum18/2
  Swing Phase/2(StimSOL) -> Mux1/2
  Demux/2 -> ANMC STIM 1/1
  Demux/1 -> "ANMC STIM "/1
  "ANMC STIM "/1 -> StimTA/1
  ANMC STIM 1/1 -> StimSOL/1

== system nmm2DFullBody/Full Body Control (created using the nmc library)/Right Side/SOL&TA Muscles/TA Actuation ==
  note: TA Actuation
  phiAnkle : Inport
  StimTA : Inport  Port=2
  " TA Muscle Spindles" : Gain  Gain=1/loptTA
  " TA loop delay" : TransportDelay  DelayTime=LongDelay
  Gain : Gain  Gain=-1
  Mux8 : Mux  Inputs=5
  Product1 : Product  RndMeth=Zero
  Saturation2 : Saturate  UpperLimit=inf  LowerLimit=0  ZeroCross=off
  Stimulation Bias3 : Constant  Value=LceOffsetTA
  Subsystem3 : nmc/Subsystem4  GotoTag=RIGHT_TA_FORCE  GotoTag2=RIGHT_TA_FORCE_LOG  GotoTag3=RIGHT_TA_FORCE_NOISE_LOG
  Subsystem5 : nmc/Subsystem4  GotoTag=RIGHT_TA_STIM  GotoTag2=RIGHT_TA_STIM_LOG  GotoTag3=RIGHT_TA_STIM_NOISE_LOG
  Subsystem6 : nmc/Subsystem4  GotoTag=RIGHT_TA_LENGTH  GotoTag2=RIGHT_TA_LENGTH_LOG  GotoTag3=RIGHT_TA_LENGTH_NOISE_LOG
  Subsystem7 : nmc/Subsystem4  GotoTag=RIGHT_TA_VELOCITY  GotoTag2=RIGHT_TA_VELOCITY_LOG  GotoTag3=RIGHT_TA_VELOCITY_NOISE_LOG
  Sum21 : Sum  Inputs=-+|  SaturateOnIntegerOverflow=on  InputSameDT=on  OutDataTypeStr=Inherit: Same as first input
  TA : Subsystem
  TA Link : Subsystem
  Terminator8 : Terminator
  LceTA : Outport
  TauTa : Outport  Port=2
  wires:
  TA/1(Fmtc) -> Subsystem3/1
  TA/2(Lce) -> Subsystem6/1
  TA/5(A) -> Mux8/5
  TA Link/1(lmtc [m]) -> TA/2(lmtc [m])
  TA Link/2(lever [m]) -> Product1/2
  " TA Muscle Spindles"/1 -> Sum21/2
  Sum21/1 -> Saturation2/1
  Mux8/1 -> Terminator8/1
  TA/4(Lse) -> Mux8/4
  TA/3(Vce) -> Subsystem7/1
  phiAnkle/1 -> TA Link/1(phi12 [rad])
  Stimulation Bias3/1 -> Sum21/1
  Saturation2/1 -> " TA loop delay"/1
  Product1/1 -> Gain/1
  StimTA/1 -> Subsystem5/1
  " TA loop delay"/1 -> LceTA/1
  Gain/1 -> TauTa/1
  Subsystem5/1 -> TA/1(STIM)
  Subsystem3/1 -> Product1/1, Mux8/1
  Subsystem6/1 -> " TA Muscle Spindles"/1, Mux8/2
  Subsystem7/1 -> Mux8/3

== system nmm2DFullBody/Full Body Control (created using the nmc library)/Right Side/VAS Muscle/VAS Actuation  ==
  note: VAS Actuation
  phiKnee : Inport
  StimVas : Inport  Port=2
  " VAS Golgi Tendon Organs" : Gain
  Gain : Gain  Gain=-1
  Mux9 : Mux  Inputs=5
  Product4 : Product  RndMeth=Zero
  Subsystem3 : nmc/Subsystem4  GotoTag=RIGHT_VAS_FORCE  GotoTag2=RIGHT_VAS_FORCE_LOG  GotoTag3=RIGHT_VAS_FORCE_NOISE_LOG
  Subsystem5 : nmc/Subsystem4  GotoTag=RIGHT_VAS_STIM  GotoTag2=RIGHT_VAS_STIM_LOG  GotoTag3=RIGHT_VAS_STIM_NOISE_LOG
  Subsystem6 : nmc/Subsystem4  GotoTag=RIGHT_VAS_LENGTH  GotoTag2=RIGHT_VAS_LENGTH_LOG  GotoTag3=RIGHT_VAS_LENGTH_NOISE_LOG
  Subsystem7 : nmc/Subsystem4  GotoTag=RIGHT_VAS_VELOCITY  GotoTag2=RIGHT_VAS_VELOCITY_LOG  GotoTag3=RIGHT_VAS_VELOCITY_NOISE_LOG
  Subsystem8 : nmc/Subsystem4  GotoTag=RIGHT_VAS_GOLGI  GotoTag2=RIGHT_VAS_GOLGI_LOG  GotoTag3=RIGHT_VAS_GOLGI_NOISE_LOG
  Terminator9 : Terminator
  VAS : Subsystem
  VAS Link : Subsystem
  VAS loop delay : TransportDelay  DelayTime=MidDelay
  TauVas : Outport
  FmVas : Outport  Port=2
  wires:
  VAS Link/1(lmtu [m]) -> VAS/2(lmtc [m])
  Product4/1 -> Gain/1
  VAS/5(A) -> Mux9/5
  VAS/1(Fmtc) -> Subsystem3/1
  VAS Link/2(lever [m]) -> Product4/1
  Mux9/1 -> Terminator9/1
  VAS/4(Lse) -> Mux9/4
  VAS/3(Vce) -> Subsystem7/1
  VAS/2(Lce) -> Subsystem6/1
  phiKnee/1 -> VAS Link/1(phi23 [rad])
  StimVas/1 -> Subsystem5/1
  Gain/1 -> TauVas/1
  " VAS Golgi Tendon Organs"/1 -> VAS loop delay/1
  VAS loop delay/1 -> FmVas/1
  Subsystem5/1 -> VAS/1(STIM)
  Subsystem3/1 -> Mux9/1, Product4/2, Subsystem8/1
  Subsystem6/1 -> Mux9/2
  Subsystem7/1 -> Mux9/3
  Subsystem8/1 -> " VAS Golgi Tendon Organs"/1

== system nmm2DFullBody/Full Body Control (created using the nmc library)/Right Side/VAS Muscle/VAS Control ==
  note: VAS Control
  FmVAS : Inport
  OLdxThigh : Inport  Port=2
  OLonCL : Inport  Port=3
  CLKneeState : Inport  Port=4
  StanceSwing : Inport  Port=5
  " Swing Phase" : Subsystem  TreatAsAtomicUnit=on
  "ANMC STIM " : Concatenate  NumInputs=1
  Logical Operator : Logic  Operator=NOT  AllPortsSameDT=off  OutDataTypeStr=boolean
  Saturation17 : Saturate  UpperLimit=1  LowerLimit=0.01  ZeroCross=off
  Stance Phase : Subsystem  TreatAsAtomicUnit=on
  Sum18 : Sum
  StimVAS : Outport
  wires:
  Logical Operator/1 -> " Swing Phase"/Enable
  FmVAS/1 -> Stance Phase/4(FmVAS)
  StanceSwing/1 -> Logical Operator/1, Stance Phase/Enable
  " Swing Phase"/1(StimVAS) -> Sum18/2
  Sum18/1 -> Saturation17/1
  Saturation17/1 -> "ANMC STIM "/1
  Stance Phase/1(StimVAS) -> Sum18/1
  OLdxThigh/1 -> Stance Phase/3(OLdxThigh [N])
  OLonCL/1 -> Stance Phase/2(OLonCL)
  CLKneeState/1 -> Stance Phase/1(CLKneeState)
  "ANMC STIM "/1 -> StimVAS/1

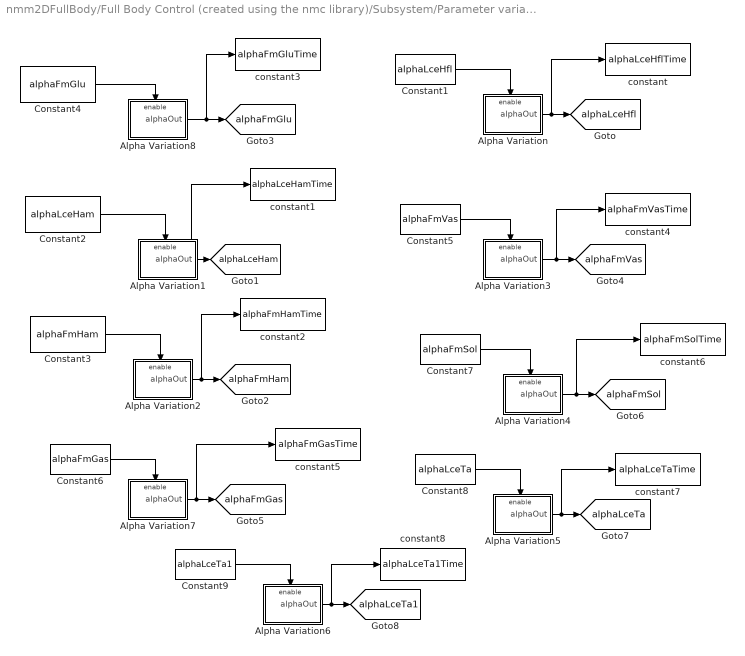
== system nmm2DFullBody/Full Body Control (created using the nmc library)/Subsystem/Parameter variation/Alpha variation ==
  Alpha Variation : Subsystem
  Alpha Variation1 : Subsystem
  Alpha Variation2 : Subsystem
  Alpha Variation3 : Subsystem
  Alpha Variation4 : Subsystem
  Alpha Variation5 : Subsystem
  Alpha Variation6 : Subsystem
  Alpha Variation7 : Subsystem
  Alpha Variation8 : Subsystem
  Constant1 : Constant  Value=alphaLceHfl
  Constant2 : Constant  Value=alphaLceHam
  Constant3 : Constant  Value=alphaFmHam
  Constant4 : Constant  Value=alphaFmGlu
  Constant5 : Constant  Value=alphaFmVas
  Constant6 : Constant  Value=alphaFmGas
  Constant7 : Constant  Value=alphaFmSol
  Constant8 : Constant  Value=alphaLceTa
  Constant9 : Constant  Value=alphaLceTa1
  constant : ToWorkspace  VariableName=alphaLceHflTime  SaveFormat=Timeseries  SampleTime=-1
  constant1 : ToWorkspace  VariableName=alphaLceHamTime  SaveFormat=Timeseries  SampleTime=-1
  constant2 : ToWorkspace  VariableName=alphaFmHamTime  SaveFormat=Timeseries  SampleTime=-1
  constant3 : ToWorkspace  VariableName=alphaFmGluTime  SaveFormat=Timeseries  SampleTime=-1
  constant4 : ToWorkspace  VariableName=alphaFmVasTime  SaveFormat=Timeseries  SampleTime=-1
  constant5 : ToWorkspace  VariableName=alphaFmGasTime  SaveFormat=Timeseries  SampleTime=-1
  constant6 : ToWorkspace  VariableName=alphaFmSolTime  SaveFormat=Timeseries  SampleTime=-1
  constant7 : ToWorkspace  VariableName=alphaLceTaTime  SaveFormat=Timeseries  SampleTime=-1
  constant8 : ToWorkspace  VariableName=alphaLceTa1Time  SaveFormat=Timeseries  SampleTime=-1
  tag scope: alphaFmGas=global, alphaFmGlu=global, alphaFmHam=global, alphaFmSol=global, alphaFmVas=global, alphaLceHam=global, alphaLceHfl=global, alphaLceTa1=global, alphaLceTa=global
  wires:
  Alpha Variation/1("alphaOut ") -> constant/1, [alphaLceHfl]
  Alpha Variation1/1("alphaOut ") -> constant1/1, [alphaLceHam]
  Alpha Variation2/1("alphaOut ") -> [alphaFmHam], constant2/1
  Constant3/1 -> Alpha Variation2/Enable
  Constant4/1 -> Alpha Variation8/Enable
  Alpha Variation8/1("alphaOut ") -> constant3/1, [alphaFmGlu]
  Constant5/1 -> Alpha Variation3/Enable
  Alpha Variation6/1("alphaOut ") -> constant8/1, [alphaLceTa1]
  Alpha Variation3/1("alphaOut ") -> constant4/1, [alphaFmVas]
  Alpha Variation7/1("alphaOut ") -> constant5/1, [alphaFmGas]
  Constant6/1 -> Alpha Variation7/Enable
  Constant7/1 -> Alpha Variation4/Enable
  Alpha Variation4/1("alphaOut ") -> constant6/1, [alphaFmSol]
  Alpha Variation5/1("alphaOut ") -> constant7/1, [alphaLceTa]
  Constant8/1 -> Alpha Variation5/Enable
  Constant9/1 -> Alpha Variation6/Enable
  Constant2/1 -> Alpha Variation1/Enable
  Constant1/1 -> Alpha Variation/Enable

== system nmm2DFullBody/Full Body Control (created using the nmc library)/Subsystem/Parameter variation/Amplitude Variation ==
  Add : Sum  Inputs=+++
  Constant1 : Constant  Value=amp_var
  Constant17 : Constant  Value=Amp
  Demux : Demux  Outputs=3
  Down : Subsystem
  "Off " : Subsystem
  Up : Subsystem
  constant10 : ToWorkspace  VariableName=ampTime  SaveFormat=Timeseries  SampleTime=-1
  tag scope: amp=global
  wires:
  Down/1("AmpDown ") -> Add/3
  Add/1 -> constant10/1, [amp]
  Demux/2 -> Up/Enable
  Demux/1 -> "Off "/Enable
  "Off "/1("Amp ") -> Add/1
  Constant1/1 -> Demux/1
  Demux/3 -> Down/Enable
  Up/1("AmpUp ") -> Add/2
  Constant17/1 -> Down/1(Amp), "Off "/1(Amp), Up/1(Amp)

== system nmm2DFullBody/Full Body Control (created using the nmc library)/Subsystem/Parameter variation/Freq variation ==
  Add : Sum  Inputs=+++
  Constant1 : Constant  Value=freq_var
  Constant17 : Constant  Value=freq
  Demux : Demux  Outputs=3
  Down : Subsystem
  "Off " : Subsystem
  Up : Subsystem
  constant10 : ToWorkspace  VariableName=freqTime  SaveFormat=Timeseries  SampleTime=-1
  tag scope: freq=global
  wires:
  Down/1("freqDown ") -> Add/3
  Add/1 -> constant10/1, [freq]
  Demux/2 -> Up/Enable
  Demux/1 -> "Off "/Enable
  "Off "/1("Amp ") -> Add/1
  Constant1/1 -> Demux/1
  Demux/3 -> Down/Enable
  Up/1("freqUp ") -> Add/2
  Constant17/1 -> Down/1("freq "), "Off "/1(freq), Up/1("freq ")

== system nmm2DFullBody/Full Body Control (created using the nmc library)/Left Side/GAS Muscle/GAS Actuation / GAS ==
  note: SOLEUS Muscle-Tendon Dynamics
  note: Excitation Contraction Coupling
  STIM : Inport
  lmtc [m] : Inport  Port=2
  1 : Product  Inputs=**  SaturateOnIntegerOverflow=on  InputSameDT=on  OutDataTypeStr=Inherit: Same as first input
  1/lslack : Gain  Gain=1/lslackGAS  SaturateOnIntegerOverflow=on  OutDataTypeStr=Inherit: Same as input  ParamDataTypeStr=Inherit: Same as input
  BE force-length relation : Subsystem
  CE force-length relation : Subsystem
  CE inverse force-velocity relation : Subsystem
  Constant : Constant  Value=lslackGAS
  ECC TransferFcn : simulink_extras/Additional Linear/Transfer Fcn (with initial outputs)  N=[1]  D=[tau 1]  Y0=preA  U0=0
      settings: AttributesFormatString=pre-activation: %<Y0>
  Fmax : Gain  Gain=FmaxGAS  SaturateOnIntegerOverflow=on  OutDataTypeStr=Inherit: Same as input  ParamDataTypeStr=Inherit: Same as input
  Fv = Fse / (A*Fce) : Product  Inputs=*/  SaturateOnIntegerOverflow=on  InputSameDT=on  OutDataTypeStr=Inherit: Same as first input
  Integrator : Integrator  InitialConditionSource=external  LowerSaturationLimit=0.05
  PE force-length relation : Subsystem
  SE force-length relation : Subsystem
  Sum : Sum  Inputs=|+-  SaturateOnIntegerOverflow=on  InputSameDT=on  OutDataTypeStr=Inherit: Same as first input
  Sum2 : Sum  Inputs=|-+  SaturateOnIntegerOverflow=on  InputSameDT=on  OutDataTypeStr=Inherit: Same as first input
  Sum3 : Sum  SaturateOnIntegerOverflow=on  InputSameDT=on  OutDataTypeStr=Inherit: Same as first input
  Sum4 : Sum  SaturateOnIntegerOverflow=on  InputSameDT=on  OutDataTypeStr=Inherit: Same as first input
  lce/lopt : Gain  Gain=1/loptGAS  SaturateOnIntegerOverflow=on  OutDataTypeStr=Inherit: Same as input  ParamDataTypeStr=Inherit: Same as input
  vmax*lopt : Gain  Gain=vmaxGAS*loptGAS  SaturateOnIntegerOverflow=on  OutDataTypeStr=Inherit: Same as input  ParamDataTypeStr=Inherit: Same as input
  Fmtc : Outport  InitialOutput=0
  Lce : Outport  Port=2  InitialOutput=0
  Vce : Outport  Port=3  InitialOutput=0
  Lse : Outport  Port=4  InitialOutput=0
  A : Outport  Port=5  InitialOutput=0
  wires:
  Integrator/1 -> Sum/2, lce/lopt/1, Lce/1  "lce"
  Sum/1 -> 1/lslack/1, Lse/1  "lse"
  lce/lopt/1 -> CE force-length relation/1(lce [lopt]), BE force-length relation/1(lce [lopt]), PE force-length relation/1(lce [lopt])
  Fv = Fse / (A*Fce)/1 -> CE inverse force-velocity relation/1(Fv[Fmax])  "fv"
  vmax*lopt/1 -> Integrator/1, Vce/1  "vce"
  lmtc [m]/1 -> Sum2/2, Sum/1  "lmtc"
  Fmax/1 -> Fmtc/1  "Fmtc"
  1/lslack/1 -> SE force-length relation/1(lse [lslack])
  SE force-length relation/1(fse [Fmax]) -> Fmax/1, Sum4/1
  Sum2/1 -> Integrator/2
  Constant/1 -> Sum2/1
  CE force-length relation/1(fce [Fmax]) -> 1/1
  Sum4/1 -> Fv = Fse / (A*Fce)/1
  PE force-length relation/1(fpe [Fmax]) -> Sum3/1
  1/1 -> Sum3/2
  BE force-length relation/1(fbe [Fmax]) -> Sum4/2
  Sum3/1 -> Fv = Fse / (A*Fce)/2
  CE inverse force-velocity relation/1(v[vmax]) -> vmax*lopt/1
  STIM/1 -> ECC TransferFcn/1
  ECC TransferFcn/1 -> A/1, 1/2

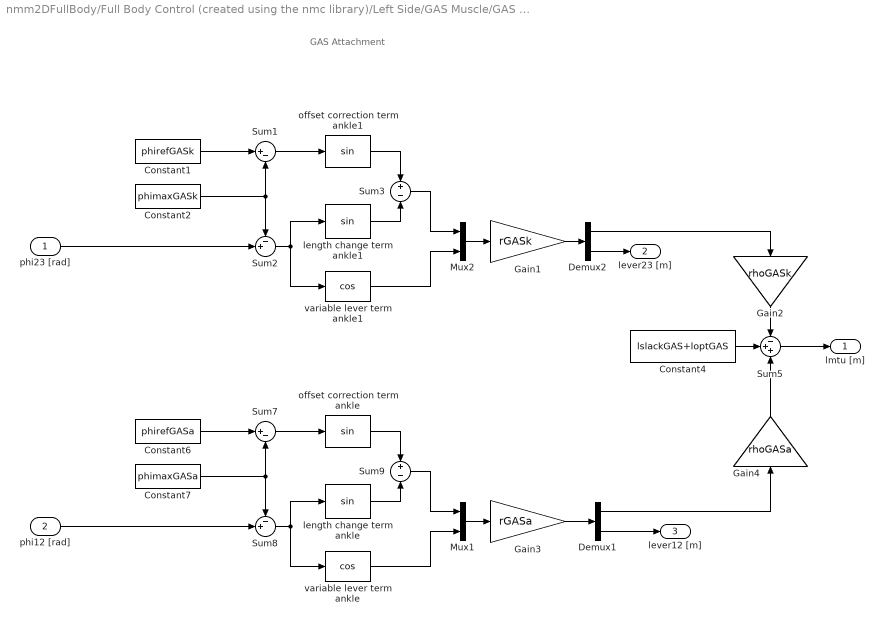
== system nmm2DFullBody/Full Body Control (created using the nmc library)/Left Side/GAS Muscle/GAS Actuation /GAS Link ==
  note: GAS Attachment
  phi23 [rad] : Inport
  phi12 [rad] : Inport  Port=2
  Constant1 : Constant  Value=phirefGASk
  Constant2 : Constant  Value=phimaxGASk
  Constant4 : Constant  Value=lslackGAS+loptGAS
  Constant6 : Constant  Value=phirefGASa
  Constant7 : Constant  Value=phimaxGASa
  Demux1 : Demux  Outputs=2
  Demux2 : Demux  Outputs=2
  Gain1 : Gain  Gain=rGASk
  Gain2 : Gain  Gain=rhoGASk
  Gain3 : Gain  Gain=rGASa
  Gain4 : Gain  Gain=rhoGASa
  Mux1 : Mux  Inputs=2
  Mux2 : Mux  Inputs=2
  Sum1 : Sum  Inputs=|+-
  Sum2 : Sum  Inputs=-+|
  Sum3 : Sum  Inputs=+-
  Sum5 : Sum  Inputs=-++
  Sum7 : Sum  Inputs=|+-
  Sum8 : Sum  Inputs=-+|
  Sum9 : Sum  Inputs=+-
  length change term ankle : Trigonometry
  length change term ankle1 : Trigonometry
  offset correction term ankle : Trigonometry
  offset correction term ankle1 : Trigonometry
  variable lever term ankle : Trigonometry  Operator=cos
  variable lever term ankle1 : Trigonometry  Operator=cos
  lmtu [m] : Outport
  lever23 [m] : Outport  Port=2
  lever12 [m] : Outport  Port=3
  wires:
  phi12 [rad]/1 -> Sum8/2
  Sum5/1 -> lmtu [m]/1
  variable lever term ankle/1 -> Mux1/2
  Demux1/2 -> lever12 [m]/1
  Sum8/1 -> variable lever term ankle/1, length change term ankle/1
  Constant7/1 -> Sum8/1, Sum7/2
  Sum7/1 -> offset correction term ankle/1
  Constant6/1 -> Sum7/1
  length change term ankle/1 -> Sum9/2
  offset correction term ankle/1 -> Sum9/1
  Sum9/1 -> Mux1/1
  Constant4/1 -> Sum5/2
  Mux1/1 -> Gain3/1
  Gain3/1 -> Demux1/1
  Demux1/1 -> Gain4/1
  Gain4/1 -> Sum5/3
  phi23 [rad]/1 -> Sum2/2
  variable lever term ankle1/1 -> Mux2/2
  Sum2/1 -> variable lever term ankle1/1, length change term ankle1/1
  Constant2/1 -> Sum2/1, Sum1/2
  Sum1/1 -> offset correction term ankle1/1
  Constant1/1 -> Sum1/1
  length change term ankle1/1 -> Sum3/2
  offset correction term ankle1/1 -> Sum3/1
  Sum3/1 -> Mux2/1
  Mux2/1 -> Gain1/1
  Gain1/1 -> Demux2/1
  Demux2/2 -> lever23 [m]/1
  Demux2/1 -> Gain2/1
  Gain2/1 -> Sum5/1

== system nmm2DFullBody/Full Body Control (created using the nmc library)/Left Side/GAS Muscle/GAS Control/ Swing Phase ==
  note: GAS Control
  note: Swing Phase Control
  Enable : EnablePort  StatesWhenEnabling=reset
  Stimulation Bias1 : Constant  Value=PreStimGAS
  StimGAS : Outport  OutputWhenDisabled=reset  InitialOutput=0
  wires:
  Stimulation Bias1/1 -> StimGAS/1

== system nmm2DFullBody/Full Body Control (created using the nmc library)/Left Side/GAS Muscle/GAS Control/Stance Phase ==
  note: GAS Control
  note: Stance Phase Control
  FmGAS : Inport
  Enable : EnablePort  StatesWhenEnabling=reset
  FB Gain2 : Gain  Gain=GainGAS  SaturateOnIntegerOverflow=on  OutDataTypeStr=Inherit: Same as input  ParamDataTypeStr=Inherit: Same as input
  Stimulation Bias1 : Constant  Value=PreStimGAS
  Sum3 : Sum  Inputs=|++  SaturateOnIntegerOverflow=on  InputSameDT=on  OutDataTypeStr=Inherit: Same as first input
  StimGAS : Outport  OutputWhenDisabled=reset  InitialOutput=0
  wires:
  FmGAS/1 -> FB Gain2/1
  Stimulation Bias1/1 -> Sum3/1
  Sum3/1 -> StimGAS/1
  FB Gain2/1 -> Sum3/2
